simulink model "new"  (R2022b)
settings: Solver=VariableStepAuto  StartTime=0.0  StopTime=1000  RelTol=1e-3
libraries: fl_lib x18, nesl_utility x11, simulink x1
settings Model: Creator=Haposan  LastModifiedBy=Haposan

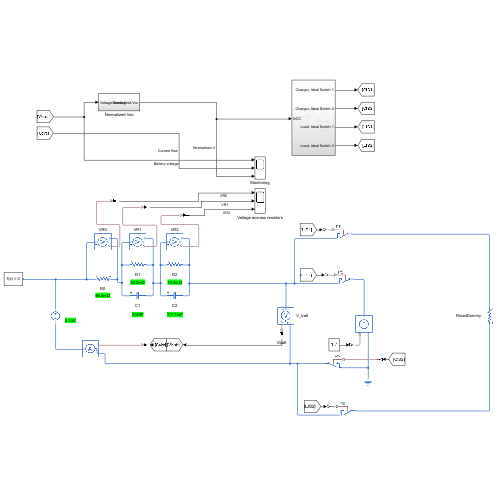
[thumbnail: Simulink's stored preview of the top-level diagram]
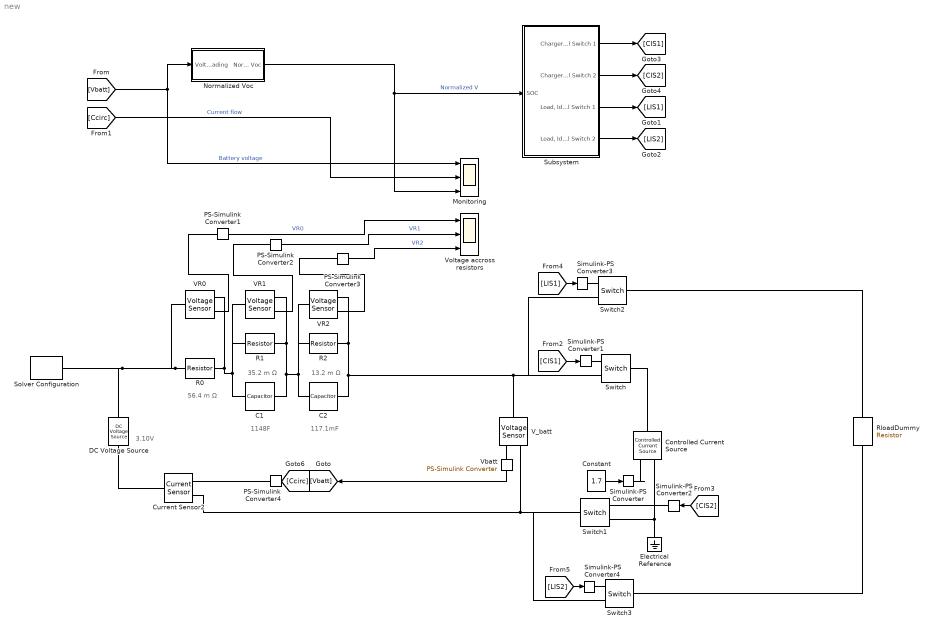
== system new ==
  note: 117.1mF
  note: 13.2 m Ω
  note: 35.2 m Ω
  note: 56.4 m Ω
  note: 1148F
  note: 3.10V
  C1 : fl_lib/Electrical/Electrical Elements/Capacitor  c=1148 F  r=1e-6 Ohm  g=0 1/Ohm  i_specify=off  i_priority=None  i=0 A  i_nominal_specify=off  i_nominal_unit=A  i_nominal_value=1  v_specify=off  v_priority=None  v=0 V  v_nominal_specify=off  v_nominal_unit=V  v_nominal_value=1  vc_specify=off  vc_priority=High  vc=0 V  vc_nominal_specify=off  vc_nominal_unit=V  vc_nominal_value=1
  C2 : fl_lib/Electrical/Electrical Elements/Capacitor  c=117.1E-3 F  r=1e-6 Ohm  g=0 1/Ohm  i_specify=off  i_priority=None  i=0 A  i_nominal_specify=off  i_nominal_unit=A  i_nominal_value=1  v_specify=off  v_priority=None  v=0 V  v_nominal_specify=off  v_nominal_unit=V  v_nominal_value=1  vc_specify=off  vc_priority=High  vc=0 V  vc_nominal_specify=off  vc_nominal_unit=V  vc_nominal_value=1
  Constant : Constant  Value=1.7
  Controlled Current Source : fl_lib/Electrical/Electrical Sources/Controlled Current Source
  Current Sensor2 : fl_lib/Electrical/Electrical Sensors/Current Sensor
  DC Voltage Source : fl_lib/Electrical/Electrical Sources/DC Voltage Source  v0=3.8 V
  Electrical Reference : fl_lib/Electrical/Electrical Elements/Electrical Reference
  Monitoring : Scope  NumInputPorts=3
  Normalized Voc : Subsystem
  PS-Simulink Converter{1..4} (4 alike) : nesl_utility/PS-Simulink Converter  PhysicalDomain=network_engine_domain  SubClassName=ps_output  LeftPortType=input  RightPortType=output  PseudoPeriodic=off  Frequencies=[]  VectorFormat=inherit  Unit=inherit  AffineConversion=off
  R0 : fl_lib/Electrical/Electrical Elements/Resistor  R=56.4E-3 Ohm  i_specify=off  i_priority=None  i=0 A  i_nominal_specify=off  i_nominal_unit=A  i_nominal_value=1  v_specify=off  v_priority=None  v=0 V  v_nominal_specify=off  v_nominal_unit=V  v_nominal_value=1
  R1 : fl_lib/Electrical/Electrical Elements/Resistor  R=35.2E-3 Ohm  i_specify=off  i_priority=None  i=0 A  i_nominal_specify=off  i_nominal_unit=A  i_nominal_value=1  v_specify=off  v_priority=None  v=0 V  v_nominal_specify=off  v_nominal_unit=V  v_nominal_value=1
  R2 : fl_lib/Electrical/Electrical Elements/Resistor  R=13.2E-3 Ohm  i_specify=off  i_priority=None  i=0 A  i_nominal_specify=off  i_nominal_unit=A  i_nominal_value=1  v_specify=off  v_priority=None  v=0 V  v_nominal_specify=off  v_nominal_unit=V  v_nominal_value=1
  RloadDummy : fl_lib/Electrical/Electrical Elements/Resistor  R=1 Ohm  i_specify=off  i_priority=None  i=0 A  i_nominal_specify=off  i_nominal_unit=A  i_nominal_value=1  v_specify=off  v_priority=None  v=0 V  v_nominal_specify=off  v_nominal_unit=V  v_nominal_value=1
  Simulink-PS Converter{,1..4} (5 alike) : nesl_utility/Simulink-PS Converter  PhysicalDomain=network_engine_domain  SubClassName=ps_input  LeftPortType=input  RightPortType=output  PseudoPeriodic=off  Frequencies=[]  NoiseDistribution=none  NoiseParameters=[]  Unit=1  AffineConversion=off  FilteringAndDerivatives=provide  SimscapeFilterOrder=1  InputFilterTimeConstant=0.001  UdotUserProvided=0
  Solver Configuration : nesl_utility/Solver Configuration  PhysicalDomain=network_engine_domain  SubClassName=solver  LeftPortType=input  RightPortType=generic  Tones=[]  Harmonics=[]  SimulateNoise=off  Profile=off  UseLocalSampling=off  EnableSwitchedLinearOptims=on  FrequencyDomain=off  UseCCode=off  RelTol=0.001  AbsTol=0.001  MinStep=1e-09  ToWorkspace=off  RevertToSquareIcSolve=off  NumHomotopyIterations=100  PhasorMode=off  PhasorModeNumHarmonics=1  ConsistencySolver=NEWTON_XTOL_AFTER_FTOL  IndexReductionMethod=DerivativeReplacement  DoDC=off  ResidualTolerance=1e-09  ConsistencyTolSource=GLOBAL  ConsistencyAbsTol=0.001  ConsistencyRelTol=0.001  ConsistencyTolFactor=0.001  UseLocalSolver=off  LocalSolverChoice=NE_BACKWARD_EULER_ADVANCER  ResolveIndetEquations=on  FunctionEvalNumThread=1  LocalSolverSampleTime=0.001  DoFixedCost=off  MaxNonlinIter=3  MaxModeIter=2  ComputeImpulses=off  ImpulseIterations=2  LinearAlgebra=auto  LinearAlgebraNumThread=0  EquationFormulation=NE_TIME_EF  DelaysMemoryBudget=1024  AutomaticFiltering=on  FilteringTimeConstant=0.001  PartitionStorageMethod=AS_NEEDED  PartitionMemoryBudget=1024  PartitionMethod=ROBUST
  Subsystem : Subsystem
  Switch{,1..3} (4 alike) : fl_lib/Electrical/Electrical Elements/Switch  R_closed=0.01 Ohm  G_open=1e-8 1/Ohm  Threshold=0.5  i_specify=off  i_priority=None  i=0 A  i_nominal_specify=off  i_nominal_unit=A  i_nominal_value=1  v_specify=off  v_priority=None  v=0 V  v_nominal_specify=off  v_nominal_unit=V  v_nominal_value=1
  VR0 : fl_lib/Electrical/Electrical Sensors/Voltage Sensor
  VR1 : fl_lib/Electrical/Electrical Sensors/Voltage Sensor
  VR2 : fl_lib/Electrical/Electrical Sensors/Voltage Sensor
  V_batt : fl_lib/Electrical/Electrical Sensors/Voltage Sensor
  Vbatt : nesl_utility/PS-Simulink Converter  PhysicalDomain=network_engine_domain  SubClassName=ps_output  LeftPortType=input  RightPortType=output  PseudoPeriodic=off  Frequencies=[]  VectorFormat=inherit  Unit=inherit  AffineConversion=off
  Voltage accross resistors : Scope  NumInputPorts=3
  wires:
  PS-Simulink Converter4/1 -> [Ccirc]
  PS-Simulink Converter3/1 -> Voltage accross resistors/3  "VR2"
  PS-Simulink Converter1/1 -> Voltage accross resistors/1  "VR0"
  PS-Simulink Converter2/1 -> Voltage accross resistors/2  "VR1"
  Vbatt/1 -> [Vbatt]
  Constant/1 -> Simulink-PS Converter/1
  Normalized Voc/1(Normalized Voc) -> Subsystem/1(SOC), Monitoring/3  "Normalized V"
  [Ccirc] -> Monitoring/2  "Current flow"
  [Vbatt] -> Normalized Voc/1(Voltage reading), Monitoring/1  "Battery voltage"
  Subsystem/2("Charger, Ideal Switch 2") -> [CIS2]
  Subsystem/1("Charger, Ideal Switch 1") -> [CIS1]
  Subsystem/3("Load, Ideal Switch 1") -> [LIS1]
  Subsystem/4("Load, Ideal Switch 2") -> [LIS2]
  [CIS1] -> Simulink-PS Converter1/1
  [CIS2] -> Simulink-PS Converter2/1
  [LIS1] -> Simulink-PS Converter3/1
  [LIS2] -> Simulink-PS Converter4/1
  connections:
  VR1/RConn2 -- C1/RConn1 -- R2/LConn1 -- VR2/LConn1 -- C2/LConn1 -- R1/RConn1
  R0/LConn1 -- DC Voltage Source/LConn1 -- Solver Configuration/RConn1 -- VR0/LConn1
  C1/LConn1 -- R1/LConn1 -- VR1/LConn1 -- VR0/RConn2 -- R0/RConn1
  VR2/RConn2 -- Switch2/RConn2 -- Switch/RConn2 -- V_batt/LConn1 -- C2/RConn1 -- R2/RConn1
  VR0/RConn1 -- PS-Simulink Converter1/LConn1
  VR2/RConn1 -- PS-Simulink Converter3/LConn1
  VR1/RConn1 -- PS-Simulink Converter2/LConn1
  PS-Simulink Converter4/LConn1 -- Current Sensor2/RConn1
  Current Sensor2/RConn2 -- Switch3/RConn2 -- Switch1/LConn1 -- V_batt/RConn2
  DC Voltage Source/RConn1 -- Current Sensor2/LConn1
  V_batt/RConn1 -- Vbatt/LConn1
  Simulink-PS Converter/RConn1 -- Controlled Current Source/RConn1
  Simulink-PS Converter1/RConn1 -- Switch/RConn1
  Switch/LConn1 -- Controlled Current Source/LConn1
  Electrical Reference/LConn1 -- Switch1/RConn2 -- Controlled Current Source/RConn2
  Simulink-PS Converter2/RConn1 -- Switch1/RConn1
  Simulink-PS Converter3/RConn1 -- Switch2/RConn1
  Simulink-PS Converter4/RConn1 -- Switch3/RConn1
  RloadDummy/LConn1 -- Switch2/LConn1
  RloadDummy/RConn1 -- Switch3/LConn1

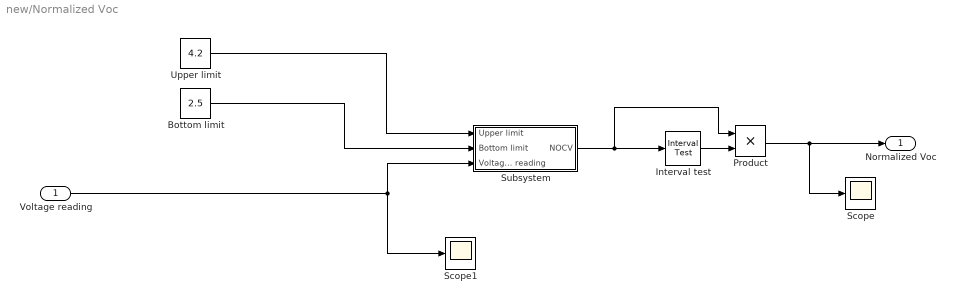
== system new/Normalized Voc ==
  Voltage reading : Inport
  Bottom limit : Constant  Value=2.5
  Interval test : simulink/Logic and Bit Operations/Interval Test  IntervalClosedRight=on  uplimit=100  IntervalClosedLeft=on  lowlimit=0  OutDataTypeStr=boolean
  Product : Product
  Scope : Scope
  Scope1 : Scope
  Subsystem : Subsystem
  Upper limit : Constant  Value=4.2
  Normalized Voc : Outport
  wires:
  Product/1 -> Scope/1, Normalized Voc/1
  Interval test/1 -> Product/2
  Subsystem/1(NOCV) -> Product/1, Interval test/1
  Bottom limit/1 -> Subsystem/2(Bottom limit)
  Voltage reading/1 -> Scope1/1, Subsystem/3(Voltage reading)
  Upper limit/1 -> Subsystem/1(Upper limit)

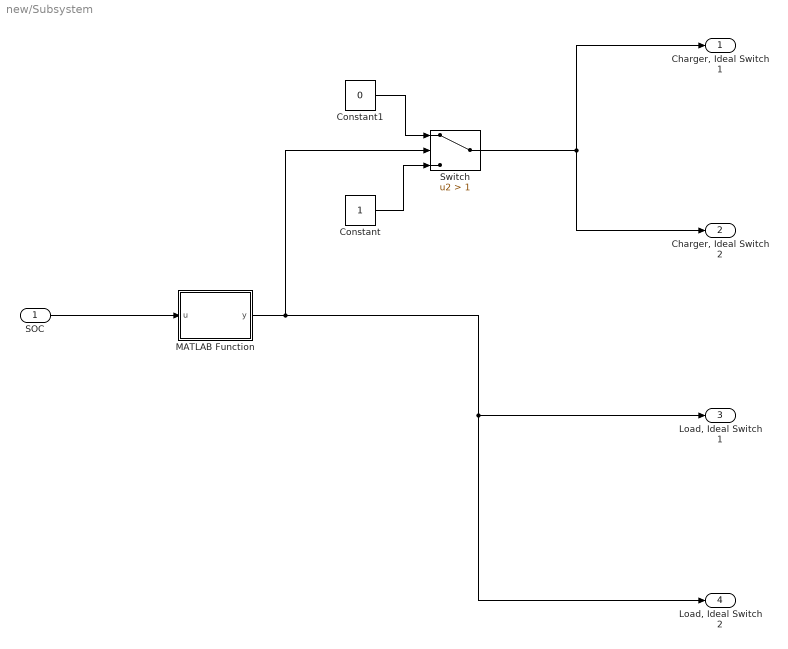
== system new/Subsystem ==
  SOC : Inport
  Constant : Constant
  Constant1 : Constant  Value=0
  MATLAB Function : MATLAB Function  TreatAsAtomicUnit=on
  Switch : Switch  Criteria=u2 > Threshold  Threshold=1  SaturateOnIntegerOverflow=off  InputSameDT=off
  "Charger, Ideal Switch 1" : Outport
  "Charger, Ideal Switch 2" : Outport  Port=2
  "Load, Ideal Switch 1" : Outport  Port=3
  "Load, Ideal Switch 2" : Outport  Port=4
  wires:
  MATLAB Function/1(y) -> Switch/2, "Load, Ideal Switch 2"/1, "Load, Ideal Switch 1"/1
  Constant1/1 -> Switch/1
  Constant/1 -> Switch/3
  SOC/1 -> MATLAB Function/1(u)
  Switch/1 -> "Charger, Ideal Switch 2"/1, "Charger, Ideal Switch 1"/1

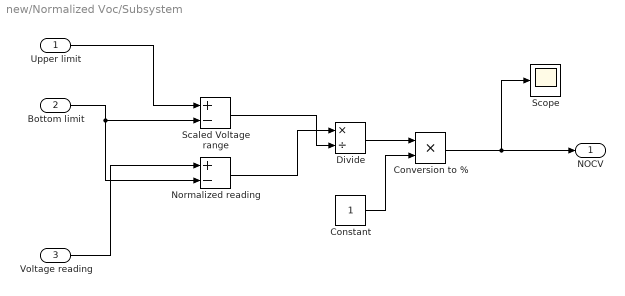
== system new/Normalized Voc/Subsystem ==
  Upper limit : Inport
  Bottom limit : Inport  Port=2
  Voltage reading : Inport  Port=3
  Constant : Constant
  Conversion to % : Product
  Divide : Product  Inputs=*/
  Normalized reading : Sum  Inputs=+-
  Scaled Voltage range : Sum  Inputs=+-
  Scope : Scope
  NOCV : Outport
  wires:
  Upper limit/1 -> Scaled Voltage range/1
  Bottom limit/1 -> Normalized reading/2, Scaled Voltage range/2
  Voltage reading/1 -> Normalized reading/1
  Normalized reading/1 -> Divide/1
  Scaled Voltage range/1 -> Divide/2
  Divide/1 -> Conversion to %/1
  Constant/1 -> Conversion to %/2
  Conversion to %/1 -> Scope/1, NOCV/1

== matlab function new/Subsystem/MATLAB Function ==
  data: u input; y output
function y = switch_output(u)
y = 1
    if u >= 99.5
        y = 1;
    elseif u <= 0
        y = 0;
    else
        y = y;  % keep the previous value of y
    end
end
